simulink model "planar_robot_ct_gravity_inertia_simulation"  (R2014a)
settings: Solver=ode45  StartTime=0.0  StopTime=10  FixedStep=0.0005  MaxStep=0.001  RelTol=1e-3
values from neighbouring files (symbols this model uses):
  a1 = u_gen(15)    [classical_joint_planar_robot_simulink.m]    (also in ct_gravit_inertia_planar_robot_simulink.m = u_gen(13); ct_gravit_planar_robot_simulink.m = u_gen(13); ct_pid_planar_robot_simulink.m; ct_planar_robot_simulink.m = u_gen(13))
  a2 = u_gen(16)    [classical_joint_planar_robot_simulink.m]    (also in ct_gravit_inertia_planar_robot_simulink.m = u_gen(14); ct_gravit_planar_robot_simulink.m = u_gen(14); ct_pid_planar_robot_simulink.m; ct_planar_robot_simulink.m = u_gen(14))
  b1 = u_gen(17)    [classical_joint_planar_robot_simulink.m]    (also in ct_gravit_inertia_planar_robot_simulink.m = u_gen(15); ct_gravit_planar_robot_simulink.m = u_gen(15); ct_pid_planar_robot_simulink.m; ct_planar_robot_simulink.m = u_gen(15))
  b2 = u_gen(18)    [classical_joint_planar_robot_simulink.m]    (also in ct_gravit_inertia_planar_robot_simulink.m = u_gen(16); ct_gravit_planar_robot_simulink.m = u_gen(16); ct_pid_planar_robot_simulink.m; ct_planar_robot_simulink.m = u_gen(16))
  g = u_gen(19)    [classical_joint_planar_robot_simulink.m]    (also in ct_gravit_inertia_planar_robot_simulink.m = u_gen(17); ct_gravit_planar_robot_simulink.m = u_gen(17); ct_pid_planar_robot_simulink.m; ct_planar_robot_simulink.m = u_gen(17))
  m1 = u_gen(11)    [ac_controller_simulink.m]    (also in classical_joint_planar_robot_simulink.m = u_gen(13); ct_gravit_inertia_planar_robot_simulink.m; ct_gravit_planar_robot_simulink.m; ct_pid_planar_robot_simulink.m = u_gen(13))
  m2 = u_gen(12)    [ac_controller_simulink.m]    (also in classical_joint_planar_robot_simulink.m = u_gen(14); ct_gravit_inertia_planar_robot_simulink.m; ct_gravit_planar_robot_simulink.m; ct_pid_planar_robot_simulink.m = u_gen(14))
settings Model: ExtModeTrigDuration=5000  Creator=Patrick  LastModifiedBy=Patrick
settings SolverCC: PositivePriorityOrder=on
settings RTWCC: SystemTargetFile=quarc_win64.tlc  TemplateMakefile=quarc_default_tmf  Description=QUARC Win64 Target  ProcessScript=quarc_win64_make_rtw_hook
settings STFCustomTargetCC: CombineOutputUpdateFcns=on  GRTInterface=off
settings GRTTargetCC: ParMdlRefBuildCompliant=off  CompOptLevelCompliant=off  MatFileLogging=off  CPPClassGenCompliant=off  ExtMode=on  ExtModeMexFile=quarc_comm

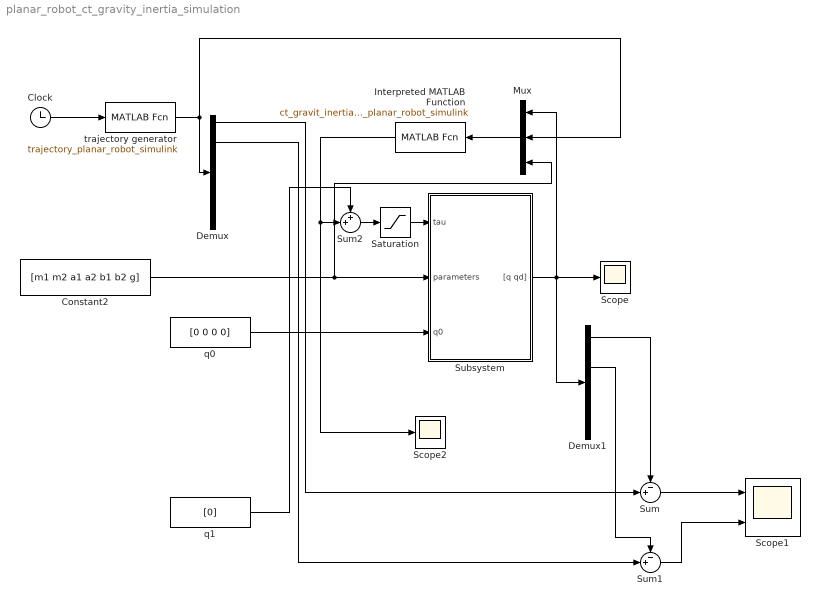
== system planar_robot_ct_gravity_inertia_simulation ==
  Clock : Clock
  Constant2 : Constant  Value=[m1 m2 a1 a2 b1 b2 g]
  Demux : Demux  Outputs=6
  Demux1 : Demux
  Interpreted MATLAB Function : MATLABFcn  MATLABFcn=ct_gravit_inertia_planar_robot_simulink
  Mux : Mux  Inputs=3
  Saturation : Saturate  UpperLimit=40  LowerLimit=-40
  Scope : Scope
      settings: YMin=-0.4  YMax=0.6
  Scope1 : Scope  NumInputPorts=2
      settings: TimeRange=10  YMin=-0.03~-2.75e-07  YMax=0.11~5e-08
  Scope2 : Scope
      settings: YMin=7.5  YMax=35  SaveName=ScopeData2
  Subsystem : Subsystem
  Sum : Sum  Inputs=-+|
  Sum1 : Sum  Inputs=-+|
  Sum2 : Sum  Inputs=++|
  q0 : Constant  Value=[0 0 0 0]
  q1 : Constant  Value=[0]
  trajectory generator : MATLABFcn  MATLABFcn=trajectory_planar_robot_simulink
  wires:
  Constant2/1 -> Mux/3, Subsystem/2(parameters)
  q0/1 -> Subsystem/3(q0)
  Subsystem/1("[q qd]") -> Demux1/1, Mux/1, Scope/1
  Mux/1 -> Interpreted MATLAB Function/1
  Clock/1 -> trajectory generator/1
  trajectory generator/1 -> Mux/2, Demux/1
  Interpreted MATLAB Function/1 -> Sum2/2, Scope2/1
  Demux/1 -> Sum/2
  Demux1/1 -> Sum/1
  Sum/1 -> Scope1/1
  Sum1/1 -> Scope1/2
  Demux1/2 -> Sum1/1
  Demux/2 -> Sum1/2
  Sum2/1 -> Saturation/1
  q1/1 -> Sum2/1
  Saturation/1 -> Subsystem/1(tau)

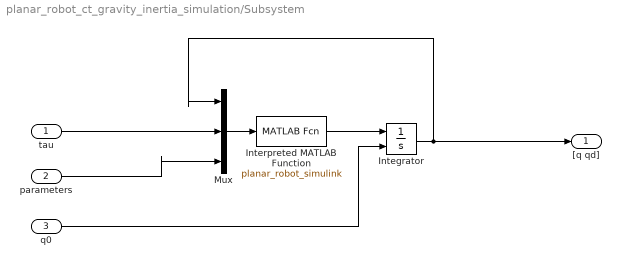
== system planar_robot_ct_gravity_inertia_simulation/Subsystem ==
  tau : Inport
  parameters : Inport  Port=2
  q0 : Inport  Port=3
  Integrator : Integrator  InitialConditionSource=external
  Interpreted MATLAB Function : MATLABFcn  MATLABFcn=planar_robot_simulink  OutputDimensions=4
  Mux : Mux  Inputs=3
  "[q qd]" : Outport
  wires:
  Interpreted MATLAB Function/1 -> Integrator/1
  tau/1 -> Mux/2
  q0/1 -> Integrator/2
  Mux/1 -> Interpreted MATLAB Function/1
  parameters/1 -> Mux/3
  Integrator/1 -> "[q qd]"/1, Mux/1
